simulink model "RateAdaptiveTrigger"  (R2018a)
settings: Solver=VariableStepAuto  StartTime=0.0  StopTime=10  RelTol=1e-3  EnableMultiTasking=on
libraries: dspswit3 x2, dspsigops x1, simulink x1
settings Model: Creator=Daniel  LastModifiedBy=Daniel
settings OptimizationCC: LifeSpan=inf
settings DebuggingCC: SFUnexpectedBacktrackingDiag=warning  SFNoUnconditionalDefaultTransitionDiag=warning  SFExecutionAtInitializationDiag=none
settings CodeAppCC: StateflowObjectComments=on
settings GRTTargetCC: TargetLangStandard=C89/C90 (ANSI)  GeneratePreprocessorConditionals=Disable all
settings ConfigComp: CovMetricSettings=dw  CovHtmlReporting=on  CovSaveCumulativeToWorkspaceVar=on  CovSaveSingleToWorkspaceVar=on  CovExternalEMLEnable=off

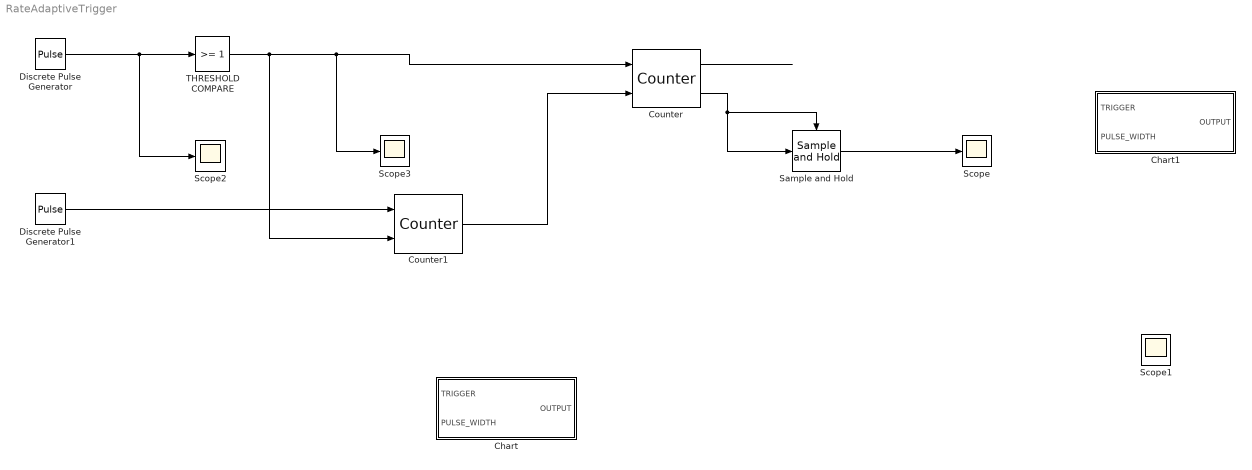
== system RateAdaptiveTrigger ==
  Chart : Stateflow chart  TreatAsAtomicUnit=on
  Chart1 : Stateflow chart  TreatAsAtomicUnit=on
  Counter : dspswit3/Counter  Direction=Up  CountEvent=Rising edge  CounterSize=User defined  MaxCount=3  InitialCount=0  Output=Count and Hit  HitValue=3  ResetInput=on  SamplesPerFrame=1  Ts=1  CntDtype=double  HitDtype=Boolean
  Counter1 : dspswit3/Counter  Direction=Up  CountEvent=Rising edge  CounterSize=User defined  MaxCount=30  InitialCount=0  Output=Hit  HitValue=30  ResetInput=on  SamplesPerFrame=1  Ts=1  CntDtype=double  HitDtype=Boolean
  Discrete Pulse Generator : DiscretePulseGenerator  Period=10  PulseWidth=2  SampleTime=0.1
  Discrete Pulse Generator1 : DiscretePulseGenerator  SampleTime=0.1
  Sample and Hold : dspsigops/Sample and Hold  trig=Rising edge  initCond=0  latchinput=off
  Scope{,1..3} (4 alike) : Scope
  THRESHOLD COMPARE : simulink/Logic and Bit Operations/Compare To Constant  relop=>=  const=1  OutDataTypeStr=boolean
  wires:
  THRESHOLD COMPARE/1 -> Counter1/2, Counter/1, Scope3/1
  Discrete Pulse Generator/1 -> Scope2/1, THRESHOLD COMPARE/1
  Counter/1 -> ?
  Discrete Pulse Generator1/1 -> Counter1/1
  Counter1/1 -> Counter/2
  Counter/2 -> Sample and Hold/Trigger, Sample and Hold/1
  Sample and Hold/1 -> Scope/1

== stateflow chart RateAdaptiveTrigger/Chart1 ==
  state PULSE_ON
    entry:
    OUTPUT=true
  state PULSE_OFF
    entry:
    OUTPUT = false
  PULSE_OFF -> PULSE_ON : after(PULSE_WIDTH, msec)
  (default) -> PULSE_ON
  PULSE_ON -> PULSE_OFF : [TRIGGER]
  data: OUTPUT output boolean =true; TRIGGER input boolean =1; PULSE_WIDTH input uint16 =10

== stateflow chart RateAdaptiveTrigger/Chart ==
  state PULSE_ON
    entry:
    OUTPUT=true
  state PULSE_OFF
    entry:
    OUTPUT = false
  PULSE_OFF -> PULSE_ON : after(PULSE_WIDTH, msec)
  (default) -> PULSE_ON
  PULSE_ON -> PULSE_OFF : [TRIGGER]
  data: OUTPUT output boolean =true; TRIGGER input boolean =1; PULSE_WIDTH input uint16 =10
